simulink model "mpc_aircraft_example"  (R2019b)
settings: Solver=ode45  StartTime=0.0  StopTime=7  RelTol=1e-3
values from neighbouring files (symbols this model uses):
  A = [-0.0151 -60.5651 0 -32.174 ... (first row only)    [UnstableAircraft.m]    (also in VincentMPCCode.m = [0 0 1 0; 0 0 0 1; -(Ks+Kus)/Mus Ks/Mus -Bs/Mus Bs/Mus; Ks/M; qpsoft.m = [           A,             minusones; scmpc4.m = [A;Su(iymax,:)]; scmpcnl2.m = [A;Su(iymax,:)])
  B = [-2.516 -13.136 ... (first row only)    [UnstableAircraft.m]    (also in VincentMPCCode.m = [0 0; 0 0; -1/Mus Kus/Mus; 1/Ms 0]; qpsoft.m = [         B; scmpc4.m = SuTQ*Su+diag(R); scmpcnl2.m = SuTQ*Su+diag(R))
  C = [0 1 0 0 ... (first row only)    [UnstableAircraft.m]    (also in VincentMPCCode.m = [1 0 0 0; -1 1 0 0; 0 0 1 0; 0 0 0 1])
  D = [0 0 ... (first row only)    [UnstableAircraft.m]    (also in VincentMPCCode.m = [0 -1; 0 0; 0 0; 0 0])
  x0 = zeros(4,1)    [UnstableAircraft.m]
libraries: mpclib x1, simulink x1
settings Model: ExtModeTrigMode=oneshot  ExtModeArmWhenConnect=off  Creator=The MathWorks, Inc.  LastModifiedBy=kieran
settings DataIOCC: SaveFormat=Array  SaveOutput=off  SignalLogging=off  DSMLogging=off  SaveTime=off  ReturnWorkspaceOutputs=off  SignalLoggingName=sigsOut
settings OptimizationCC: BooleanDataType=off  ExpressionDepthLimit=2147483647  InitFltsAndDblsToZero=on  LifeSpan=inf
settings DebuggingCC: SaveWithParameterizedLinksMsg=none  UnderspecifiedInitializationDetection=Classic  MergeDetectMultiDrivingBlocksExec=none  CheckExecutionContextPreStartOutputMsg=on  CheckExecutionContextRuntimeOutputMsg=on  SignalResolutionControl=TryResolveAllWithWarning  MultiTaskDSMMsg=warning  MultiTaskCondExecSysMsg=none  IntegerOverflowMsg=none  FcnCallInpInsideContextMsg=warning  StateNameClashWarn=warning  SFUnexpectedBacktrackingDiag=warning  SFNoUnconditionalDefaultTransitionDiag=warning  SFExecutionAtInitializationDiag=none  IntegerSaturationMsg=none  ArithmeticOperatorsInVariantConditions=warning
settings HardwareCC: ProdBitPerPointer=32  ProdBitPerSizeT=32  ProdBitPerPtrDiffT=32  ProdLargestAtomicFloat=None  ProdIntDivRoundTo=Undefined  ProdEndianess=Unspecified  ProdWordSize=32  ProdHWDeviceType=32-bit Generic  TargetUnknown=on
settings ModelReferenceCC: PropagateSignalLabelsOutOfModel=off
settings SFSimCC: SimUseLocalCustomCode=off  CustomCodeUndefinedFunction=UseInterfaceOnly
settings RTWCC: RTWUseLocalCustomCode=off
settings CodeAppCC: StateflowObjectComments=on
settings GRTTargetCC: TargetFcnLib=ansi_tfl_tmw.mat  TargetLangStandard=C89/C90 (ANSI)  GeneratePreprocessorConditionals=Disable all  CombineOutputUpdateFcns=off  GRTInterface=on
settings ConfigComp: CovMetricSettings=dw  CovHtmlReporting=on  CovSaveCumulativeToWorkspaceVar=on  CovSaveSingleToWorkspaceVar=on  CovExternalEMLEnable=off  CovSFcnEnable=off

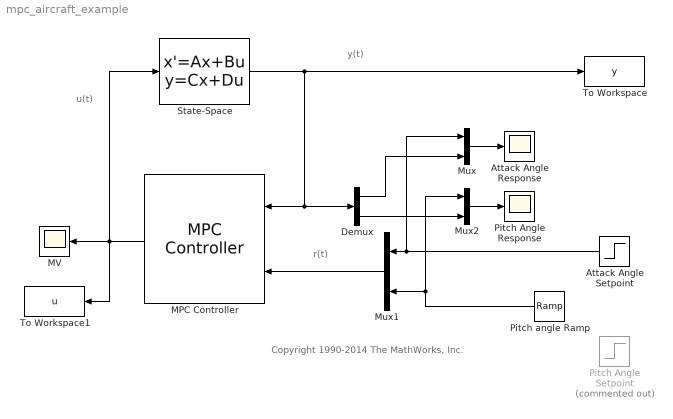
== system mpc_aircraft_example ==
  note: u(t)
  note: y(t)
  note: r(t)
  note: Copyright 1990-2014 The MathWorks, Inc.
  Attack Angle Response : Scope
  Attack Angle Setpoint : Step  Time=4  After=0.1  SampleTime=0
  Demux : Demux  Outputs=2
  MPC Controller : mpclib/MPC Controller  mpcobj=mpcobj  x0=[]  is_multiple=0  enable_value=0  return_u0=off  updateMPCinCallerWorkspace=on  md_inport=off  mv_inport=off  uref_inport=off  return_cost=off  return_mvseq=off  return_qpstatus=off  return_xseq=off  return_state=off  return_ovseq=off  state_inport=off  umin_inport=off  umax_inport=off  ymin_inport=off  ymax_inport=off  cc_inport=off  ywt_inport=off  uwt_inport=off  duwt_inport=off  rhoeps_inport=off  pm_inport=off  MaximumP=10  HorizonChoice=FixedHorizon  n_ts=0.05  n_p=10  n_mv=2  n_md=0  n_ud=0  n_mo=2  n_uo=0  BlockDataType=double  SampleTimeInherited=off  switch_inport=off
  MV : Scope
  Mux : Mux  Inputs=2
  Mux1 : Mux  Inputs=2
  Mux2 : Mux  Inputs=2
  Pitch Angle Response : Scope
  Pitch Angle Setpoint : Step  Commented=on  After=10  SampleTime=0
  Pitch angle Ramp : simulink/Sources/Ramp  slope=10/7  start=0  InitialOutput=0
  State-Space : StateSpace  A=A  B=B  C=C  D=D  InitialCondition=x0
  To Workspace : ToWorkspace  VariableName=y  SampleTime=-1
  To Workspace1 : ToWorkspace  VariableName=u  SampleTime=-1
  wires:
  State-Space/1 -> To Workspace/1, MPC Controller/1, Demux/1
  Mux/1 -> Attack Angle Response/1
  MPC Controller/1 -> To Workspace1/1, State-Space/1, MV/1
  Attack Angle Setpoint/1 -> Mux/1, Mux1/1
  Pitch angle Ramp/1 -> Mux2/1, Mux1/2
  Mux1/1 -> MPC Controller/2
  Demux/1 -> Mux/2
  Mux2/1 -> Pitch Angle Response/1
  Demux/2 -> Mux2/2
